simulink library "etherlab_lib_exp"  (Simulink 6.4)
undefined symbols (not defined in the file or in its folder): Address, catch_check
(part 2 of 3)

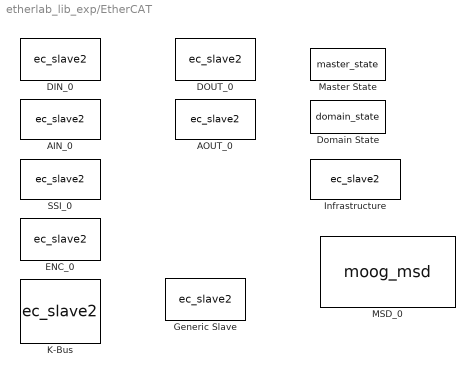
== system etherlab_lib_exp/EtherCAT ==
  AIN_0 : S-Function  FunctionName=ec_slave2  Parameters=Address,SlaveConfig,LayoutVersion,SdoConfig,output,tsample  mask(EL31xx){master=0, index=1, model=EL3102, output_type=Vector Output, scale=1, offset=0, dtype=Double, status=off, filter=off, tau=0.1, tsample=0}
      mask prompts: index "Slave Index"; model "Device Model"; output_type "Output Type"; scale "Output Full Scale"; offset "Output Offset"; dtype "Output Data Type"; status "Status Output"; filter "Output Filter"; tau "LPF Time Constant (sec)"; tsample "Sample Time"
      mask help:
      | Beckhoff 2,4,8-Channel 16-Bit Analog Input
      |
      | Output Type:
      |   1-Byte output: one bit coded input
      |   Vector output: Output vector is <Channels> wide
      |   Separate outputs: have <Channels> number of outputs
      |
      | Input Gain/Offset:
      |   Specify a possible Gain and Offset for the input signal
      mask init:
      | masterStr = '';
      | positionStr = '';
      | [Address masterStr positionStr] = getEtherCATAddress(gcb,master,index);
      | 
      | SdoConfig = [];
      | 
      | % Find the product code from the available models
      | models = struct(...
      |     'EL3102'  ,{{hex2dec('0C1E3052') 0 '-10..10V'}}, ...
      |     'EL3152'  ,{{hex2dec('0C503052') 0 '4..20mA'}}, ...
      |     'EL3162'  ,{{hex2dec('0C5A3052') 0 '0-10V'}} ...  
      |     );
      | 
      | if isfield(models,model)
      |     selection = models.(model);
      | else
      |     errordlg([gcb ': Slave model "' model '" is not implemented'])
      | end
      | 
      | func = selection{3};
      | 
      | EtherCATInfoFile = 'EtherCATInfo_el3xxx';
      | try 
      |     load(EtherCATInfoFile);
      | catch
      |     errordlg([gcb ': Could not load EtherCATInfo MAT file '...
      |         'EtherCATInfo_el3xxx']);
      |     % Regenerate with: 
      |     %  EtherCATInfo_el3xxx = getEtherCATInfo('Beckhoff EL3xxx.xml')
      |     %  save EtherCATInfo_el3xxx 'EtherCATInfo_el3xxx'
      | end
      | LayoutVersion = 0;
      | 
      | output = [];
      | 
      | device = EtherCATInfo_el3xxx(selection{1},selection{2});
      | if isempty(device)
      |     errordlg(sprintf(...
      |         ['%s: Could not find device with\n'...
      |         'ProductCode \t#x%08X\n'...
      |         'RevisionNo \t#x%08X\n'...
      |         'in file %s.'],...
      |         gcs, selection{1}, selection{2}, EtherCATInfoFile));
      | else
      |     channels = str2double(model(6));
      |     if status
      |         StatusPdoEntries = [12544 + (1:channels); ones(1,channels)]';
      |         PdoEntries = [12544 + (1:channels); 1 + ones(1,channels)]';
      |     else
      |         PdoEntries = [25600 + ones(1,channels); 1:channels]';
      |     end
      | 
      |     SlaveConfig = genSlaveConfig(device,EtherCATInfo_el3xxx.VendorId);
      |     PdoEntryMap = generateIO(device);
      |     if output_type == 1
      |         % Vector output chosen
      | 
      |         output(1).PdoEntry = PdoEntries;
      | 
      |         if status
      |             output(2).PdoEntry = StatusPdoEntries;
      |         end
      | 
      |         if dtype ~= 1
      |              output(1).PdoFullScale = 2^15;
      | 
      |             if dtype == 3
      |                 output(1).Gain = scale;
      |                 output(1).Offset = offset;
      |                 output(1).GainName = 'FullScale';
      |                 output(1).OffsetName = 'Offset';
      |             end
      |             if filter
      |                 if sum(tau == 0)
      |                     errordlg([gcb ': Specify a nonzero time constant '...
      |                         'for the output filter.']);
      |                 end
      |                 if (tsample)
      |                     output(1).Filter = tsample./tau;
      |                     output(1).FilterName = 'InputWeight';
      |                 else
      |                     output(1).Filter = 2*pi./tau;
      |                     output(1).FilterName = 'Omega';
      |                 end
      |             end
      |         end
      | 
      |     else
      |         % Separate outputs chosen
      |         % Distribute each row of output_pdo_map to output(x).pdo_map
      |         output = cell2struct(mat2cell(PdoEntries,ones(1,channels),2),'PdoEntry',2);
      |         if status
      |             output = [output; ...
      |                 cell2struct(mat2cell(StatusPdoEntries,ones(1,channels),2),'PdoEntry',2)];
      |         end
      | 
      |         if dtype ~= 1
      |             for i = 1:channels
      |                 output(i).PdoFullScale = 2^15;
      |             end
      | 
      |             if dtype == 3
      |                 if ~isempty(scale)
      |                     for i = 1:channels
      |                         % Choose scale(1) for every output if scale
      |                         % is a scalar
      |                         output(i).Gain = scale(min(i,max(size(scale))));
      |                         output(i).GainName = ['FullScale' num2str(i)];
      |                     end
      |                 end
      | 
      |                 if ~isempty(offset)
      |                     for i = 1:channels
      |                         % Choose offset(1) for every output if offset
      |                         % is a scalar
      |                         output(i).Offset = offset(min(i,max(size(offset))));
      |                         output(i).OffsetName = ['Offset' num2str(i)];
      |                     end
      |                 end
      |             end
      | 
      |             if filter && ~isempty(tau)
      |                 if sum(tau == 0)
      |                     errordlg([gcb ': Specify a nonzero time constant '...
      |                         'for the output filter.']);
      |                 end
      | 
      |                 if tsample(1)
      |                     k = tsample(1)./tau;
      |                     prefix = 'InputWeight';
      |                 else
      |                     k = 2*pi./tau;
      |                     prefix = 'Omega';
      |                 end
      |                 for i = 1:channels
      |                     % Choose k(1) for every output if k
      |                     % is a scalar
      |                     output(i).Filter = k(min(i,max(size(k))));
      |                     output(i).FilterName = [prefix num2str(i)];
      |                 end
      | 
      |             end
      |         end
      |     end
      | end
      mask Help:
      | This block generically implements the EtherCAT 16-Bit Analog Input Terminal for various models.
      | <p/>
      | The following Terminals are supported:
      | <center>
      | <table width="80%">
      | <tr><td>EL3102,4,8</td><td>-10..10V Voltage Input</td></tr>
      | <tr><td>EL3112,4   </td><td>0..20mA Current Input</td></tr>
      | <tr><td>EL3122,4   </td><td>4..20mA Current Input</td></tr>
      | <tr><td>EL3142,4,8</td><td>0..20mA Current Input</td></tr>
      | <tr><td>EL3152,4,8</td><td>4..20mA Current Input</td></tr>
      | <tr><td>EL3162,4,8</td><td>0..10V Voltage Input</td></tr>
      | </table>
      | </center>
      | <p/>
      | Choose and set the following options:
      | <h4>Master:</h4>
      | Set the EtherCAT Master of this terminal.
      | 
      | <h4>Slave Index:</h4>
      | Set the EtherCAT slave index. Following address formats are allowed:
      | <ol>
      | <li> Absolute addressing: a number <<b><tt>n</tt></b>> representing the (zero based) absolute index. <b><tt>n</tt></b> is typically larger than 0 because the first coupler has that address.
      | 
      | <li> Field addressing: Has the form <<b><tt>f:n</tt></b>> where <b><tt>f</tt></b> is the (zero based) EtherCAT coupler field and
      | <b><tt>n</tt></b> is the terminal offset in that field. Take note that <b><tt>n</tt></b> is also greater than 0.
      | 
      | <li> SSId addressing: the Secondary Slave Addressing has the form <<b><tt>#s:n</tt></b>> where <b><tt>s</tt></b> is the Secondary Slave Id of the EtherCAT coupler and <b><tt>n</tt></b> is the offset in that field. The SSId has to be preprogrammed into the coupler with other service tools.
      | </ol>
      | 
      | <h4>Device Model:</h4>
      | Choose the model at the Indexed position of the master.
      | 
      | <h4>Output Type:</h4>
      | <ul>
      | <li>Choose <b>Vector Output</b> to have a single output as a vector
      | with a size corresponding to the channel count of the terminal. This mode also allows a status output port to be displayed. <br/>
      | <li>Choose <b>Separate Outputs</b> to have one output for every channel.
      | </ul>
      | <h4>Output Full Scale</h4>
      | When <b>Output Data Type</b> is set to <b>Double with scale and offset</b>, the block's output value at full scale terminal input can be set here.
      | 
      | <h4>Output Offset</h4>
      | When <b>Output Data Type</b> is set to <b>Double with scale and offset</b>, the blocks output at zero terminal input can be set here. Note that the Full Scale above is also increased by this amount. Note furthermore that this corresponds to the minimum input for terminals such as 4..20mA.
      | 
      | <h4>Output Data Type</h4>
      | Choose the block's output data type for the output signal. Available are:
      | <ul>
      | <li><b><tt>Raw</tt></b> outputting the internal raw value as <tt>int16_T</tt> or <tt>uint16_T</tt> as appropriate
      | <li><b><tt>Double</tt></b> outputting 0..10, -10..10, 0..0.02 and 0.004..0.02 depending on the Model as appropriate
      | <li><b><tt>Double with scale and offset</tt></b>, allowing the output to be scaled with an offset.
      | </ul>
      | 
      | <p>
      | Choosing <b>Status Output</b> provides a port of type <tt>uint8_T</tt> where the status is presented. This is only enabled when <b>Vector Output</b> is selected. Terminal input over- and underrange can be detected using this output. See the terminal's documentation.
      | 
      | <h4>Output Filter</h4>
      | When not in <b>Raw</b> mode, the <b>Output Filter</b> checkbox becomes available, allowing the use of an internal low pass filter. Enter the <b>LPF Time Constant</b> for the filter in the field below.
      | <br>For continuous sample time systems (0 in Sample Time), the filter is also continuous. Discrete samples systems (Sample Time > 0) uses an equivalent discrete low pass filter with a similar time constant.
      | 
      | <p>
      | Set the <b>Sample Time</b> for the block. <tt>0</tt> is continuous sample time (runs at the model's base rate). Setting <tt>-1</tt> will try to set the time using back propagation.
      mask StyleString: edit,edit,popup(EL3102|EL3152|EL3162),popup(Vector Output|Separate Outputs),edit,edit,popup(Raw bits|Double|Double with scale and offset),checkbox,checkbox,edit,edit
      mask CallbackString:
      | |||el31xx_check('output_type');
      | |||el31xx_check('dtype');||el31xx_check('filter');||
      mask Display:
      | fprintf('%s\n%s AIn\nM:%s Idx:%s',...
      |     model,func,masterStr,positionStr)
  AOUT_0 : S-Function  FunctionName=ec_slave2  Parameters=Address,SlaveConfig,LayoutVersion,SdoConfig,input,tsample  mask(EL41xx){master=0, index=1, model=EL4102, input_type=Vector Input, scale=[], tsample=-1}
      mask prompts: index "Slave Index"; model "Device Model"; input_type "Input Type"; scale "Input Full Scale (empty for none)"; tsample "Sample Time (-1 for inherited)"
      mask help:
      | Beckhoff 2,4,8-Channel 16-Bit Analog Output
      |
      | Input Type:
      |   1-Byte input: one bit coded input
      |   Vector input: Input vector is <Channels> wide
      |   Separate inputs: have <Channels> number of inputs
      mask init:
      | masterStr = '';
      | positionStr = '';
      | [Address masterStr positionStr] = getEtherCATAddress(gcb,master,index);
      | 
      | SdoConfig = [];
      | 
      | % Find the product code from the available models
      | models = struct(...
      |     'EL4102'  ,{{hex2dec('10063052') 0                   '0..10V' }}, ...
      |     'EL4132'  ,{{hex2dec('10243052') hex2dec('F0000000') '+-10V'  }}, ...
      |     'EL4132v2',{{hex2dec('10243052') 0                   '+-10V'  }}, ...
      |     'EL4122'  ,{{hex2dec('101a3052') 0                   '4..20mA'}},...  
      |     'EL4112'  ,{{hex2dec('10103052') 0                   '0..20mA'}} ...  
      |     );
      | 
      | SdoConfig = [];
      | 
      | if isfield(models,model)
      |     selection = models.(model);
      | else
      |     errordlg([gcb ': Slave model "' model '" is not implemented'])
      | end
      | 
      | func = selection{3};
      | 
      | EtherCATInfoFile = 'EtherCATInfo_el4xxx';
      | try 
      |     load(EtherCATInfoFile);
      | catch
      |     errordlg([gcb ': Could not load EtherCATInfo MAT file '...
      |         'EtherCATInfo_el4xxx']);
      |     % Regenerate with: 
      |     %  EtherCATInfo_el4xxx = getEtherCATInfo('Beckhoff EL4xxx.xml')
      |     % Note that in this case you will not have Rev #xF0000000 for
      |     % EL4132 then, unless you create one yourself
      | end
      | 
      | LayoutVersion = 0;
      | 
      | device = EtherCATInfo_el4xxx(selection{1},selection{2});
      | input = [];
      | if isempty(device)
      |     errordlg(sprintf(...
      |         ['%s: Could not find device with\n'...
      |         'ProductCode \t#x%08X\n'...
      |         'RevisionNo \t#x%08X\n'...
      |         'in file %s.'],...
      |         gcs, selection{1}, selection{2}, EtherCATInfoFile));
      | else
      |     SlaveConfig = genSlaveConfig(device, EtherCATInfo_el4xxx.VendorId);
      |     % Number of channels is given by the 6'th character of model string
      |     channels = str2double(model(6));
      | 
      |     input = [];
      |     if input_type == 1
      |         PdoEntryMap = generateIO(device, 'GroupType', 'All');
      |         input = cell2struct(PdoEntryMap,'PdoEntry',1);
      |         input.PdoFullScale = 2^15;
      |         if ~isempty(scale)
      |             input.Gain = scale;
      |             input.GainName = 'FullScale';
      |         end
      |     elseif input_type == 2
      |         PdoEntryMap = generateIO(device);
      |         fs = repmat({2^15},1,channels);
      |         input = struct('PdoEntry', PdoEntryMap, 'PdoFullScale', 2^15);
      |         if ~isempty(scale)
      |             for i = 1:channels
      |                 input(i).Gain = scale(min(i,max(size(scale))));
      |                 input(i).GainName = ['FullScale' num2str(i)];
      |             end
      |         end
      |     end
      | end
      mask Help:
      | This block generically implements the EtherCAT 16-Bit Analog Input Terminal for various models.
      | <p/>
      | The block input is generally a <tt>double</tt> corresponding the the terminal's capability. Thus a 4..20mA terminal expects values in the range [0.004..0.02). If a digital input is required, only <tt>uint16</tt> or <tt>int16</tt> is accepted, depending on whether the the terminal is bipolar or not.
      | <p/>
      | Exceeding the input range simply saturates the terminal's output.
      | <p/>
      | The following Terminals are supported:
      | <center>
      | <table width="80%">
      | <tr><td>EL4102,4,8</td><td>0..10V Voltage Output</td></tr>
      | <tr><td>EL4112,4,8</td><td>0..20mA Current Output</td></tr>
      | <tr><td>EL4122,4,8</td><td>4..20mA Current Output</td></tr>
      | <tr><td>EL4132,4,8</td><td>-10..10V Voltage Output</td></tr>
      | </table>
      | </center>
      | <p/>
      | Choose and set the following options:
      | <h4>Master:</h4>
      | Set the EtherCAT Master of this terminal.
      | 
      | <h4>Slave Index:</h4>
      | Set the EtherCAT slave index. Following address formats are allowed:
      | <ol>
      | <li> Absolute addressing: a number <<b><tt>n</tt></b>> representing the (zero based) absolute index. <b><tt>n</tt></b> is typically larger than 0 because the first coupler has that address.
      | 
      | <li> Field addressing: Has the form <<b><tt>f:n</tt></b>> where <b><tt>f</tt></b> is the (zero based) EtherCAT coupler field and
      | <b><tt>n</tt></b> is the terminal offset in that field. Take note that <b><tt>n</tt></b> is also greater than 0.
      | 
      | <li> SSId addressing: the Secondary Slave Addressing has the form <<b><tt>#s:n</tt></b>> where <b><tt>s</tt></b> is the Secondary Slave Id of the EtherCAT coupler and <b><tt>n</tt></b> is the offset in that field. The SSId has to be preprogrammed into the coupler with other service tools.
      | </ol>
      | 
      | <h4>Device Model:</h4>
      | Choose the device at the Indexed position of the master.
      | 
      | <h4>Input Type:</h4>
      | <ul>
      | <li>Choose <b>Vector Input</b> to have a single input as a vector
      | with a size corresponding to the channel count of the terminal. This mode also allows a control input and a status output port to be displayed.
      | <li>Choose <b>Separate Inputs</b> to have one input for every channel.
      | </ul>
      | 
      | <p>
      | Choosing <b>Status Output</b> provides a port of type <tt>uint8_T</tt> where the status is presented. This is only enabled when <b>Vector Output</b> is selected. Note: at the time of writing (1.2.2006) the terminals do not have a status output, and hence this option is disabled!
      | 
      | <p>
      | Set the <b>Sample Time</b> for the block. <tt>0</tt> is continuous sample time (runs at the model's base rate). Setting <tt>-1</tt> will try to set the time using back propagation.
      mask StyleString: edit,edit,popup(EL4102|EL4112|EL4122|EL4132v2|-- Obsolete|EL4132),popup(Vector Input|Separate Inputs),edit,edit
      mask Display:
      | fprintf('%s\n%s AIn\nM:%s Idx:%s',...
      |     model,func,masterStr,positionStr)
  DIN_0 : S-Function  FunctionName=ec_slave2  Parameters=Address,SlaveConfig,LayoutVersion,SdoConfig,IOSpec,tsample  mask(EL10xx){master=0, index=1, model=EL1004v2, output_type=Vector Output, tsample=0}
      mask prompts: index "Slave Index"; model "Device Model"; output_type "Output Type"; tsample "Sample Time"
      mask help:
      | Beckhoff EtherCAT Digital Input
      | EL1002,4,8:	3ms filter
      | EL1012,4,8:	10us filter
      | EL1004v2: Newer version with PDO at 0x6000
      |
      | Output Type:
      |   1-Byte output: one bit coded output
      |   Vector output: Output vector is <Channels> wide
      |   Separate outputs: have <Channels> number of outputs
      mask init:
      | masterStr = '';
      | positionStr = '';
      | [Address masterStr positionStr] = getEtherCATAddress(gcb,master,index);
      | 
      | SdoConfig = [];
      | 
      | % Find the product code from the available models
      | models = struct(...
      |     'EL1004'  ,[hex2dec('03ec3052')     hex2dec('0010000A')], ...
      |     'EL1004v2',[hex2dec('03ec3052')     hex2dec('00100000')], ...
      |     'EL1008'  ,[hex2dec('03f03052')     hex2dec('00100000')], ...
      |     'EL1014v2',[hex2dec('03f63052')     hex2dec('00100000')], ...  
      |     'EL1014'  ,[hex2dec('03f63052')     hex2dec('00000000')], ...  
      |     'EL1018'  ,[hex2dec('03fa3052')     hex2dec('00100000')]  ...
      |     );
      | 
      | if isfield(models,model)
      |     selection = models.(model);
      | else
      |     errordlg([gcb ': Slave model "' model '" is not implemented'])
      | end
      | 
      | EtherCATInfoFile = 'EtherCATInfo_el1xxx';
      | try 
      |     load(EtherCATInfoFile);
      | catch
      |     errordlg([gcb ': Could not load EtherCATInfo MAT file '...
      |         'EtherCATInfo_el1xxx']);
      |     % Regenerate with: 
      |     %  EtherCATInfo_el1xxx = getEtherCATInfo('Beckhoff EL1xxx.xml')
      |     %  save EtherCATInfo_el1xxx
      | end
      | 
      | LayoutVersion = 0;
      | 
      | IOSpec = [];
      | 
      | device = EtherCATInfo_el1xxx(selection(1),selection(2));
      | if isempty(device)
      |     errordlg(sprintf(...
      |         ['%s: Could not find device with\n'...
      |         'ProductCode \t#x%08X\n'...
      |         'RevisionNo \t#x%08X\n'...
      |         'in file %s.'],...
      |         gcs, selection(1), selection(2), EtherCATInfoFile));
      | else
      |     
      |     SlaveConfig = ...
      |         genSlaveConfig(device,EtherCATInfo_el1xxx.VendorId);
      |     
      |     if strcmp(output_type, 'Vector Output')
      |         % Only one output, with all rows of pdo_map
      |         PdoEntryMap = generateIO(device, 'GroupType', 'All');
      |         IOSpec = cell2struct(PdoEntryMap,'PdoEntry',1);
      | 
      |     elseif strcmp(output_type, 'Separate Outputs')
      |         % Have (channel) number of outputs, each containing one row of pdo_map
      |         PdoEntryMap = generateIO(device);
      |         IOSpec = cell2struct(PdoEntryMap,'PdoEntry',1);
      |     else
      |         errordlg([gcb ': unknown output type: ' output_type]);
      |         IOSpec = [];
      |     end
      | end
      mask Help:
      | This block implements the Beckhoff's EtherCAT series of Digital Input Terminals.
      | <p/>
      | Choose or set the following options:
      | <h4>Master:</h4>
      | Set the EtherCAT Master number that this terminal is connected to.
      | 
      | <h4>Slave Index:</h4>
      | Set the EtherCAT slave index. Following address formats are allowed:
      | <ol>
      | <li> Absolute addressing: a number <<b><tt>n</tt></b>> representing the (zero based) absolute index. <b><tt>n</tt></b> is typically larger than 0 because the first coupler has that address.
      | 
      | <li> Field addressing: Has the form <<b><tt>f:n</tt></b>> where <b><tt>f</tt></b> is the (zero based) EtherCAT coupler field and
      | <b><tt>n</tt></b> is the terminal offset in that field. Take note that <b><tt>n</tt></b> is also greater than 0.
      | 
      | <li> SSId addressing: the Secondary Slave Addressing has the form <<b><tt>#s:n</tt></b>> where <b><tt>s</tt></b> is the Secondary Slave Id of the EtherCAT coupler and <b><tt>n</tt></b> is the offset in that field. The SSId has to be preprogrammed into the coupler with other service tools.
      | </ol>
      | 
      | <h4> Device Model</h4>
      | Select the model that is used. This sets the number of outputs of this block.
      | 
      | <h4>Output Type</h4>
      | The block output type corresponding to the terminal inputs can be one of the following:
      | <ul>
      | <li><b>1-Byte Output</b>: This sets one output where each digital input to the terminal occupies one bit.
      | <li><b>Vector Output</b>: This sets one output vector with a width equal to the number of digital inputs to the terminal.
      | <li><b>Separate Outputs</b>: This sets the number of outputs corresponding to the digital inputs to the terminal.
      | </ul>
      | 
      | <h4>Output Data Type</h4>
      | Select the output data type that is required.
      | 
      | <h4>Sample Time</h4>
      | Select the correct sample time. Setting this to 0 makes for a sample time at the model's base rate. If another block can set the sample time, choose -1 for inherited sample time.
      mask StyleString: edit,edit,popup(EL1004v2|EL1008|EL1014v2|EL1018|-- Obsolete|EL1004|EL1014),popup(Vector Output|Separate Outputs),edit
      mask Display:
      | fprintf('%s\nM:%s Idx:%s',...
      |     model,'',positionStr)
  DOUT_0 : S-Function  FunctionName=ec_slave2  Parameters=Address,SlaveConfig,LayoutVersion,SdoConfig,IOSpec,tsample  mask(EL20xx){master=0, index=1, model=EL2004v2, input_type=Vector Input, status=off, tsample=0}
      mask prompts: index "Slave Index"; model "Device Model"; input_type "Input Type"; status "Status Output"; tsample "Sample Time (-1 for inherited)"
      mask help:
      | Beckhoff EtherCAT Digital Output
      | EL2002,4:	24V 0.5A
      | EL2032:		24V 2A, Optional Status (with Vector Input)
      |
      | Input Type:
      |   1-Byte input: one bit coded input
      |   Vector input: Input vector is <Channels> wide
      |   Separate inputs: have <Channels> number of inputs
      mask init:
      | masterStr = '';
      | positionStr = '';
      | [Address masterStr positionStr] = getEtherCATAddress(gcb,master,index);
      | 
      | SdoConfig = [];
      | 
      | % Find the product code from the available models
      | models = struct(...
      |     'EL2004'  ,[hex2dec('07d43052')  hex2dec('00000000')], ...
      |     'EL2004v2',[hex2dec('07d43052')  hex2dec('00100000')], ...
      |     'EL2008'  ,[hex2dec('07d83052')  hex2dec('00100000')], ...
      |     'EL2032'  ,[hex2dec('07f03052')  hex2dec('00000000')], ...
      |     'EL2032v2',[hex2dec('07f03052')  hex2dec('00100000')], ...
      |     'EL2602'  ,[hex2dec('0a2a3052')  hex2dec('00100000')], ...
      |     'EL2612'  ,[hex2dec('0a343052')  hex2dec('00100000')], ...
      |     'EL2622'  ,[hex2dec('0a3e3052')  hex2dec('00100000')]  ...
      |     );
      | 
      | if isfield(models,model)
      |     selection = models.(model);
      | else
      |     errordlg([gcb ': Slave model "' model '" is not implemented'])
      | end
      | 
      | LayoutVersion = 0;
      | 
      | try 
      |     load EtherCATInfo_el2xxx;
      | catch
      |     errordlg([gcb ': Could not load EtherCATInfo MAT file '...
      |         'EtherCATInfo_el2xxx']);
      |     % Regenerate with: 
      |     %  EtherCATInfo_el2xxx = getEtherCATInfo('Beckhoff EL2xxx.xml')
      |     %  save EtherCATInfo_el2xxx 'EtherCATInfo_el2xxx'
      | end
      | 
      | IOSpec = [];
      | 
      | device = EtherCATInfo_el2xxx(selection(1),selection(2));
      | if isempty(device)
      |     errordlg(sprintf(...
      |         ['%s: Could not find device with\n'...
      |         'ProductCode \t#x%08X\n'...
      |         'RevisionNo \t#x%08X\n'...
      |         'in file "%s".'],...
      |         gcs, selection(1), selection(2), 'EtherCATInfo_el2xxx'));
      | else
      |     SlaveConfig = genSlaveConfig(device,EtherCATInfo_el2xxx.VendorId);
      |     
      |     channels = str2double(model(6));
      |     PdoIndexList = hex2dec('1600') + [0:channels-1];
      |     if status
      |         PdoIndexList = [PdoIndexList  hex2dec('1A00') + [0:channels-1]];
      |     end
      | 
      |     if strcmp(input_type,'Vector Input')
      |         % Only one output, with all rows of pdo_map
      |         PdoEntryMap = generateIO(device, 'GroupType', 'All',...
      |             'SelectPdo', PdoIndexList);
      |         IOSpec = cell2struct(PdoEntryMap,'PdoEntry',1);
      |     elseif strcmp(input_type, 'Separate Inputs')
      |         % Have (channel) number of outputs, each containing one row of pdo_map
      |         PdoEntryMap = generateIO(device);
      |         IOSpec = cell2struct(PdoEntryMap,'PdoEntry',1);
      |     else
      |         errordlg([gcb ': unknown input type: ' input_type]);
      |     end
      | end
      mask Help:
      | This block implements the Beckhoff's EtherCAT series of Digital Output Terminals.
      | <p/>
      | Choose or set the following options:
      | <h4>Master:</h4>
      | Set the EtherCAT Master number that this terminal is connected to.
      | 
      | <h4>Slave Index:</h4>
      | Set the EtherCAT slave index. Following address formats are allowed:
      | <ol>
      | <li> Absolute addressing: a number <<b><tt>n</tt></b>> representing the (zero based) absolute index. <b><tt>n</tt></b> is typically larger than 0 because the first coupler has that address.
      | 
      | <li> Field addressing: Has the form <<b><tt>f:n</tt></b>> where <b><tt>f</tt></b> is the (zero based) EtherCAT coupler field and
      | <b><tt>n</tt></b> is the terminal offset in that field. Take note that <b><tt>n</tt></b> is also greater than 0.
      | 
      | <li> SSId addressing: the Secondary Slave Addressing has the form <<b><tt>#s:n</tt></b>> where <b><tt>s</tt></b> is the Secondary Slave Id of the EtherCAT coupler and <b><tt>n</tt></b> is the offset in that field. The SSId has to be preprogrammed into the coupler with other service tools.
      | </ol>
      | 
      | <h4> Device Model</h4>
      | Select the model that is used. This sets the maximum number of inputs of this block. Having fewer inputs is allowed.<br>
      |  Some models have an optional status byte. These have the <b>Status Output</b> below enabled.
      | 
      | <h4>Input Type</h4>
      | The input type can be one of the following:
      | <ul>
      | <li><b>1-Byte Input</b>: This sets one block input bit coded corresponding to the digital output of the terminal.
      | <li><b>Vector Input</b>: This sets one input vector where each element corresponds to a digital output of the terminal.
      | <li><b>Separate Inputs</b>: This sets the number of block inputs corresponding to the digital output count of the terminal.
      | </ul>
      | 
      | <h4>Status Output</h4>
      | Some models have a status bit to monitor the attached hardware. Check this box to make it available as a block output in simulink. This option is not available if <b>Separate Inputs</b> is selected.
      | 
      | <h4>Sample Time</h4>
      | Select the correct sample time. Setting this to 0 makes for a sample time at the model's base rate. If another block can set the sample time, choose -1 for inherited sample time.
      mask StyleString: edit,edit,popup(EL2004v2|EL2008|EL2032v2|EL2602|EL2612|EL2622|-- Obsolete|EL2004|EL2032),popup(Vector Input|Separate Inputs),checkbox,edit
      mask CallbackString:
      | ||status_idx = find(strcmp(get_param(gcb,'MaskNames'),'status'));
      | 
      | en = get_param(gcb,'MaskEnables');
      | 
      | if findstr('2032',get_param(gcb,'model'))
      |         en{status_idx} = 'on';
      | else
      |     en{status_idx} = 'off';
      | end
      | set_param(gcb,'MaskEnables',en);
      | |||
      mask Display:
      | fprintf('%s\nM:%s Idx:%s',...
      |     model,masterStr,positionStr)
  Domain State : S-Function  FunctionName=domain_state  Parameters=master,domain,input,output,tsample  mask(Domain State){master=0, domain=0, direction=Input Only, tsample=0}
      mask prompts: tsample "Sample Time"
      mask help:
      | Displays the following domain state information:
      | * Working Counter
      | * Domain state:
      | 	0 - No slaves
      | 	1 - Domain incomplete
      | 	2 - Domain complete
      mask init:
      | switch direction
      |     case 1
      |         input = 1;
      |         output = 0;
      |     case 2
      |         input = 0;
      |         output = 1;
      |     case 3
      |         input = 1;
      |         output = 1;
      | end
      mask StyleString: edit,edit,popup(Input Only|Output Only|Input and Output),edit
      mask Display:
      | fprintf('Domain State\nM:%u d:%u',
      | master,domain);
  ENC_0 : S-Function  FunctionName=ec_slave2  Parameters=Address,SlaveConfig,LayoutVersion,SdoConfig,IOSpec,tsample  mask(EL5101){master=0, index=1, reload=off, reset=off, fwdcount=off, gate=None, freqwin=100, reloadvalue=65535, control=off, preset=off, dtype=Double, value=on, latch=off, freq=off, period=off, window=off, status=off, tsample=0}
      mask prompts: index "Slave Index"; reload "Enable Register Reload"; reset "Enable Index Reset"; fwdcount "Enable FWD Count"; freqwin "Frequency Window (0..65535)"; reloadvalue "Counter Reload Value (0..65535)"; control "Control Input Port"; preset "Preset Input Port"; dtype "Output Data Type"; value "Counter Value Output Port"; latch "Latch Output Port"; freq "Frequency Output Port"; period "Period Output Port"; window "Window Output Port"; status "Status Output Port"; tsample "Sample Time (-1 inherited)"
      mask help: Beckhoff EtherCAT Incremental Encoder Input
      mask init:
      | masterStr = '';
      | positionStr = '';
      | [Address masterStr positionStr] = getEtherCATAddress(gcb,master,index);
      | 
      | product_code = hex2dec('13ed3052');
      | revision_no = hex2dec('00010000');
      | LayoutVersion = 0;
      | 
      | try 
      |     load EtherCATInfo_el5xxx
      | catch
      |     errordlg([gcb ': Could not load EtherCATInfo MAT file '...
      |         'EtherCATInfo_el5xxx']);
      |     % Regenerate with: 
      |     %  EtherCATInfo_el5xxx = getEtherCATInfo('Beckhoff EL5xxx.xml')
      |     %  save EtherCATInfo_el5xxx 'EtherCATInfo_el5xxx'
      | end
      | SlaveConfig = genSlaveConfig(EtherCATInfo_el5xxx, product_code, revision_no);
      | 
      | 
      | % PDO Entry is a definition of all PDO's that exist in the slave
      | % List here a matrix, where every row has 3 elements:
      | % 1: PDO index
      | % 2: PDO subindex
      | % 3: Bit size (8,16,32); Negative values mean signed values
      | pdo_entry = struct(...
      |     'status' , [hex2dec('6000'), 1], ...
      |     'value'  , [hex2dec('6000'), 2], ...
      |     'latch'  , [hex2dec('6000'), 3], ...
      |     'freq'   , [hex2dec('6000'), 4], ...
      |     'period' , [hex2dec('6000'), 5], ...
      |     'window' , [hex2dec('6000'), 6], ...
      |     'control', [hex2dec('7000'), 1], ...
      |     'preset' , [hex2dec('7000'), 2]);
      | 
      | 
      | % SDO Config is the configuration of a slave
      | % It is a matrix, every row having 4 elements:
      | % 1: SDO Index
      | % 2: SDO Subindex
      | % 3: Size    (8,16,32)
      | % 4: value
      | SdoConfig = [
      |     hex2dec('8000'), 1,  8, reloadvalue == 1;... % Reload
      |     hex2dec('8000'), 2,  8, reset == 1      ;... % Index Reset
      |     hex2dec('8000'), 3,  8, fwdcount == 1   ;... % Forward Count
      |     hex2dec('8000'), 4,  8, gate == 2       ;... % Positive Gate
      |     hex2dec('8000'), 5,  8, gate == 3       ;... % Negative Gate
      |     hex2dec('8001'), 1, 16, freqwin         ;... % Frequency Window
      |     hex2dec('8001'), 2, 16, reloadvalue     ;... % Reload Value
      |     ];
      | SdoConfig = cell2struct(...
      |     num2cell(SdoConfig),...
      |     {'Index' 'SubIndex' 'BitLen' 'Value'}, 2);
      | 
      | % This maps ???
      | % It is a matrix, every row having 4 elements:
      | % 1: PDO direction as seen by the slave: 0 = output; 1 = Input
      | % 2: PDO Index
      | % 3: Starting row of PDO entry (Zero based)
      | % 4: Number of PDO entry rows
      | IOSpec = [];
      | if ~isempty(SlaveConfig)
      |     port = 1;
      |     if value
      |         IOSpec(port).PdoEntry = pdo_entry.value;
      |         if dtype == 2
      |             IOSpec(port).PdoFullScale = 2^16;
      |         end
      | 
      |         port = port + 1;
      |     end
      |     if latch
      |         IOSpec(port).PdoEntry = pdo_entry.latch;
      |         if dtype == 2
      |             IOSpec(port).PdoFullScale = 2^16;
      |         end
      | 
      |         port = port + 1;
      |     end
      |     if freq
      |         IOSpec(port).PdoEntry = pdo_entry.freq;
      |         if dtype == 2
      |             IOSpec(port).PdoFullScale = 2^32;
      |         end
      | 
      |         port = port + 1;
      |     end
      |     if period
      |         IOSpec(port).PdoEntry = pdo_entry.period;
      |         if dtype == 2
      |             IOSpec(port).PdoFullScale = 2^16;
      |         end
      | 
      |         port = port + 1;
      |     end
      |     if window
      |         IOSpec(port).PdoEntry = pdo_entry.window;
      |         if dtype == 2
      |             IOSpec(port).PdoFullScale = 2^16;
      |         end
      | 
      |         port = port + 1;
      |     end
      |     if status
      |         IOSpec(port).PdoEntry = pdo_entry.status;
      | 
      |         port = port + 1;
      |     end
      | 
      |     if control
      |         IOSpec(port).PdoEntry = pdo_entry.control;
      | 
      |         port = port + 1;
      |     end
      |     if preset
      |         IOSpec(port).PdoEntry = pdo_entry.preset;
      |         if dtype == 2
      |             IOSpec(port).PdoFullScale = 2^16;
      |         end
      | 
      |         port = port + 1;
      |     end
      | end
      mask Help:
      | This block implements the EtherCAT Incremental Encoder Input Terminal EL5101.
      | 
      | The first output is data, the second optional output is a Status Byte. Various options affect the behaviour of the terminal and the block's output:
      | 
      | <h4>Master:</h4>
      | Set the EtherCAT Master of this terminal.
      | 
      | <h4>Slave Index:</h4>
      | Set the EtherCAT slave index. Following address formats are allowed:
      | <ol>
      | <li> Absolute addressing: a string '<b><tt>n</tt></b>' representing the (zero based) absolute index. <b><tt>n</tt></b> is typically larger than 0 because the first coupler has that address.
      | 
      | <li> SSId addressing: the Secondary Slave Addressing has the form '<b><tt>#s:n</tt></b>' where <b><tt>s</tt></b> is the Secondary Slave Id of the EtherCAT coupler and <b><tt>n</tt></b> is the offset in that field. The SSId has to be preprogrammed into the coupler with other service tools.
      | </ol>
      | 
      | <h4>Configuration Parameters</h4>
      | <dl>
      | <dt><b><tt>Enable Register Reload</tt></b></dt>
      | <dd>When the counter value wraps (either overflows or underflows), reload the value specified in <em>Counter Reload Value</em>. This option cannot be used together with <em>Enable Index Reset</em></dd>
      | 
      | <dt><b><tt>Enable Index Reset</tt></b></dt>
      | <dd>activates terminal input "C", which resets the counter value. This option cannot be used together with <em>Enable Register Reload</em>.</dd>
      | 
      | <dt><b><tt>Enable FWD Count</tt></b></dt>
      | <dd>disables quadrature evaluation of the "A" and "B" terminal inputs. Counter only counts up.</dd>
      | 
      | <dt><b><tt>Gate</tt></b></dt>
      | <dd>
      | Stops the counter on either <b>Rising</b> or <b>Falling</b> edge. This input is enabled when <em>Latch Output Port</en> is enabled.
      | </dd>
      | 
      | <dt><b><tt>Frequency Window</tt></b></dt>
      | <dd>Value determines the width of the Window variable in increments of 16us (whatever that means???) This input is enabled when <em>Frequency Output Port</em> is selected</dd>
      | 
      | <dt><b><tt>Counter Reload Value</tt></b></dt>
      | <dd>The value with which the counter is reloaded in case of <em>Enable Register Reload</em> is activated</dd>
      | </dl>
      | 
      | <h4>Inputs</h4>
      | Enable <tt><b>Control Input Port</b></tt> or <tt><b>Preset Input Port</b></tt>. Refer to the documentation for these rather complex inputs. The ordering of the inputs matches the ordering in the configuration mask.
      | 
      | <h4>Output Data Type</h4>
      | Choose the block's output data type for the output signal. Available are:
      | <ul>
      | <li><b><tt>Raw</tt></b> outputting the internal raw value as <tt>uint32_T</tt> as appropriate
      | <li><b><tt>Double</tt></b> outputting 0..1 corresponding to the Full Scale. Full Scale is affected by the Frame Type, SSI Frame Size and Data Length. Refer to manufactuer's documentation.
      | </ul>
      | 
      | <h4>Outputs</h4>
      | Select the desired outputs as presented int the configuratoin mask. The ordering matches the ordering in the mask. Refer to manufacturors documentation.
      | 
      | <p>
      | Set the <b>Sample Time</b> for the block. <tt>0</tt> is continuous sample time (runs at the model's base rate). Setting <tt>-1</tt> will try to set the time using back propagation.
      mask StyleString: edit,edit,checkbox,checkbox,checkbox,popup(None|Positive|Negative),edit,edit,checkbox,checkbox,popup(Raw bits|Double),checkbox,checkbox,checkbox,checkbox,checkbox,checkbox,edit
      mask CallbackString: ||el5101_check('Reload');|el5101_check('IndexReset');|||||||||el5101_check('Latch');|el5101_check('Freq');||||
      mask Display:
      | fprintf('EL5101\nIncr.-Enc\nM:%s Idx:%s',...
      |     masterStr, positionStr)
  Generic Slave : S-Function  FunctionName=ec_slave2  Parameters=Address,SlaveConfig,LayoutVersion,SdoConfig,IOSpec,tsample  mask(Generic EtherCAT Slave){master=0, index=1, ethercatinfo='', product_code=hex2dec('0'), revision=[], pdo_list=[], group=No Grouping, sdo_config=[], tsample=0}
      mask prompts: index "Slave Index"; ethercatinfo "EtherCATInfo XML file"; product_code "Product Code"; revision "Revision (empty for latest)"; pdo_list "Mapped PDO (empty for all)"; group "Group PDO Entries"; sdo_config "SDO Config"; tsample "Sample Time (-1 inherited)"
      mask help: Implements a generic EtherCAT Slave as described in the EtherCATInfo XML File
      mask init:
      | masterStr = '';
      | positionStr = '';
      | product_name = 'Unknown';
      | [Address masterStr positionStr] = getEtherCATAddress(gcb,master,index);
      | 
      | SdoConfig = [];
      | 
      | % Generate a LayoutVersion that is unique for every slave
      | % of this type to enure that a separate slave config is generated
      | % for every slave
      | LayoutVersion = 0;
      | 
      | try
      |     fname = char(ethercatinfo);
      | catch
      |     errordlg([gcb ':File name for EtherCAT Info not a valid string']);
      | end
      | 
      | if ~(isnumeric(product_code) && isnumeric(revision) ...
      |         && isnumeric(pdo_list) && isnumeric(sdo_config))
      |     fname = '';
      |     errordlg([gcb ':Value for Product Code, Revision Number '...
      |         'Pdo List and Sdo Config must be numeric']);
      | end
      |     
      | IOSpec = [];
      | SlaveConfig = [];
      | 
      | if isempty(fname)
      |     IOSpec = [];
      |     SlaveConfig = [];
      | elseif isempty(dir(fname))
      |     warndlg([gcb ':File ''' fname ''' not found']);
      | else
      |     switch lower(group)
      |         case 'group data types in pdo'
      |             type = 'PDO';
      |         case 'group data types'
      |             type = 'ALL';
      |         otherwise
      |             type = 'None';
      |     end
      |     ei = EtherCATInfo(fname);
      |     if ~isempty(product_code) && product_code
      |         dev = ei(product_code,revision);
      |     else
      |         dev = ei{1};
      |     end
      |     SlaveConfig = genSlaveConfig(dev, ei.VendorId);
      |     PdoEntries = generateIO(dev,'GroupType',type);
      |     if ~isempty(SlaveConfig)
      |         product_name = SlaveConfig.Type;
      |     end
      |     IOSpec = struct('PdoEntry', PdoEntries);
      | end
      mask StyleString: edit,edit,edit,edit,edit,edit,popup(No Grouping|Group Data Types in PDO|Group Data Types),edit,edit
      mask Display:
      | fprintf('%s\nM:%s Idx:%s',...
      |     product_name,masterStr,positionStr);
  Infrastructure : S-Function  FunctionName=ec_slave2  Parameters=Address,SlaveConfig,LayoutVersion,SdoConfig,output,tsample  mask(Infrastructure Block){master=0, index=0, model=EK1100, tsample=0}
      mask prompts: index "Slave Index"; model "Device Model"; tsample "Sample Time (-1 inherited)"
      mask help:
      | EtherCAT Infrastructure Slaves.
      |
      | The following slaves are available:
      | EK1100	'EtherCAT Coupler
      | EK1110	EtherCAT Extension
      | EL9110	24V w. Diag.
      | EL9160	230V w. Diag.
      | EL9210	24V w. Fuse & Diag.
      | EL9260	230V w. Fuse & Diag.
      |
      | Including these slaves (even if they don't have outputs)
      | in the bus configuration will cause them to go into the
      | operational mode
      mask init:
      | masterStr = '';
      | positionStr = '';
      | [Address masterStr positionStr] = getEtherCATAddress(gcb,master,index);
      | 
      | SdoConfig = [];
      | func = 'Unknown';
      | 
      | % Find the product code from the available models
      | models = struct( ...
      |     'EK1100', {{hex2dec('044c2c52') hex2dec('00000000') 'EtherCAT Coupler'    }}, ...
      |     'EK1110', {{hex2dec('04562c52') hex2dec('00000000') 'EtherCAT Extension'  }}, ...
      |     'EL9110', {{hex2dec('23963052') hex2dec('00100000') '24V w. Diag.'        }}, ...
      |     'EL9160', {{hex2dec('23c83052') hex2dec('00100000') '230V w. Diag.'       }}, ...
      |     'EL9210', {{hex2dec('23fa3052') hex2dec('00100000') '24V w. Fuse & Diag.' }}, ...
      |     'EL9260', {{hex2dec('242c3052') hex2dec('00100000') '230V w. Fuse & Diag.'}} ...
      |     );
      | 
      | if isfield(models,model)
      |     selection = models.(model);
      |     func = selection{3};
      | else
      |     errordlg([gcb ': Slave model "' model '" is not implemented'])
      | end
      | 
      | try
      |     switch model(1:2)
      |         case 'EK'
      |             EtherCATInfoFile = 'EtherCATInfo_ekxxxx';
      |             load(EtherCATInfoFile);
      |             ei = EtherCATInfo_ekxxxx;
      |         case 'EL'
      |             EtherCATInfoFile = 'EtherCATInfo_el9xxx';
      |             load(EtherCATInfoFile);
      |             ei = EtherCATInfo_el9xxx;
      |     end
      | catch
      |     errordlg([gcb ': Could not load EtherCATInfo MAT file ' EtherCATInfoFile]);
      | end
      | LayoutVersion = 0;
      | 
      | output = [];
      | dev = ei(selection{1}, selection{2});
      | SlaveConfig = genSlaveConfig(dev,ei.VendorId);
      | if ~isempty(dev)
      |     PdoEntries = generateIO(dev);
      |     output = struct('PdoEntry',PdoEntries);
      | end
      mask StyleString: edit,edit,popup(EK1100|EK1110|EL9110|EL9160|EL9210|EL9260),edit
      mask Display:
      | fprintf('%s\n%s\nM:%s Idx:%s',...
      |     model,func,masterStr,positionStr)
  K-Bus : S-Function  FunctionName=ec_slave2  Parameters=Address,SlaveConfig,LayoutVersion,SdoConfig,IOSpec,tsample  mask(K-Bus Coupler){master=0, index=1, ethercatinfo='', group=Group Data Types in PDO, tsample=0}
      mask prompts: index "Slave Index"; ethercatinfo "EtherCATInfo XML file"; group "Group Pdo Entries"; tsample "Sample Time (-1 inherited)"
      mask help:
      | Beckhoff EK1110 K-Bus to EtherCAT Coupler
      |
      | Group Pdo Entries:
      |   * Data Types in PDO: This option groups all Pdo Entries in a
      | 	PDO with the same data type together
      |   * All Data Types: All Pdo Entries with the same data typ
      | 	are grouped together.
      mask init:
      | masterStr = '';
      | positionStr = '';
      | display_name = '';
      | [Address masterStr positionStr] = getEtherCATAddress(gcb,master,index);
      | 
      | SdoConfig = [];
      | 
      | % Generate a LayoutVersion that is unique for every slave
      | % of this type to enure that a separate slave config is generated
      | % for every slave
      | LayoutVersion = Address.Domain * 2^16 + Address.Position;
      | 
      | fname = '';
      | 
      | try
      |     fname = char(ethercatinfo);
      | catch
      |     errordlg([gcb ':File name for EtherCAT Info not a valid string']);
      | end
      |     
      | IOSpec = [];
      | SlaveConfig = [];
      | 
      | if isempty(fname)
      |     IOSpec = [];
      |     SlaveConfig = [];
      | elseif isempty(dir(fname))
      |     warndlg([gcb ':File ''' fname ''' not found']);
      | else
      |     switch lower(group)
      |         case 'group data types in pdo'
      |             type = 'PDO';
      |         case 'group data types'
      |             type = 'ALL';
      |         otherwise
      |             type = 'None';
      |     end
      |     
      |     ei = EtherCATInfo(fname);
      |     SlaveConfig = genSlaveConfig(ei{1},ei.VendorId);
      |     PdoEntries = generateIO(ei{1},'GroupType',type);
      |     IOSpec = struct('PdoEntry', PdoEntries);
      | 
      |     [p f e] = fileparts(fname);
      |     display_name = [f e];
      | end
      mask Help:
      | This block provides an interface to the K-Bus process image for the EK1120 Coupler.
      | <p>
      | Choose and set the following options:
      | <h4>Master:</h4>
      | Set the EtherCAT Master of this terminal.
      | 
      | <h4>Slave Index:</h4>
      | Set the EtherCAT slave index. Following address formats are allowed:
      | <ol>
      | <li> Absolute addressing: a string '<b><tt>n</tt></b>' representing the (zero based) absolute index. <b><tt>n</tt></b> is typically larger than 0 because the first coupler has that address.
      | 
      | <li> SSId addressing: the Secondary Slave Addressing has the form '<b><tt>#s:n</tt></b>' where <b><tt>s</tt></b> is the Secondary Slave Id of the EtherCAT coupler and <b><tt>n</tt></b> is the offset in that field. The SSId has to be preprogrammed into the coupler with other service tools.
      | </ol>
      | 
      | <h4>EtherCATInfo XML File:</h4>
      | A string path pointing to the XML description of the k-Bus Coupler
      | 
      | <h4>Sample Time:</h4>
      | Set the <b>Sample Time</b> for the block. <tt>0</tt> is continuous sample time (runs at the model's base rate). Setting <tt>-1</tt> will try to set the time using back propagation.
      mask StyleString: edit,edit,edit,popup(No Grouping|Group Data Types in PDO|Group Data Types),edit
      mask Display:
      | fprintf('BK1120\nK-Bus Coupler\n%s\nM:%s Idx:%s',...
      |     display_name,masterStr,positionStr);
  MSD_0 : S-Function  FunctionName=moog_msd  Parameters=master,index,tsample,iomode  mask(Moog MSC){master=0, index=0, tsample=0, iomode=Inputs and Outputs}
      mask prompts: index "Slave Index"; tsample "Sample Time"; iomode "Input/Output Mode"
      mask help: Moog Servodrive Controller
      mask init:
      | moog_msd_callback('display_callback',gcb)
      mask StyleString: edit,edit,edit,popup(Inputs and Outputs|Inputs only|Outputs only)
      mask CallbackString: |||moog_msd_callback('display_callback',gcb)
      mask Display: fprintf('Moog Servo Drive\nM:%i Idx:%s', master, index) image(imread('moog.png'), [.3, .7, .4, .2]) port_label('input', 1, 'control') port_label('input', 2, 'v_tgt') port_label('output', 1, 'status') port_label('output', 2, 'v_cur')
  Master State : S-Function  FunctionName=master_state  Parameters=master,tsample  mask(Master State){master=0, tsample=0}
      mask prompts: tsample "Sample Time"
      mask help:
      | Outputs master state:
      | * number of responding slaves
      | * Slave states
      | * Link up
      mask Display:
      | fprintf('Master State\nM: %u',
      | master);
  SSI_0 : S-Function  FunctionName=ec_slave2  Parameters=Address,SlaveConfig,LayoutVersion,SdoConfig,output,tsample  mask(EL5001){master=0, index=1, scale=1, offset=0, dtype=Double, code=Binary, baud=1250k, frame=Multiturn (25 bits), fsize=25, length=24, frame_error=off, inhibit=off, inh_time=1, status=off, filter=off, tau=0.1, tsample=0}
      mask prompts: index "Slave Index"; scale "Output Full Scale"; offset "Output Offset"; dtype "Output Data Type"; code "SSI Code"; baud "Baudrate"; frame "Frame Type"; fsize "SSI Frame Size"; length "Data Length"; frame_error "Disable Frame Error"; inhibit "Enable Inhibit Time"; inh_time "Min Inhibit Time [us] (1..65535)"; status "Status Output"; filter "Output Filter"; tau "LPF Time Constant (sec)"; tsample "Sample Time"
      mask help: Beckhoff EtherCAT SSI Input
      mask init:
      | masterStr = '';
      | positionStr = '';
      | [Address masterStr positionStr] = getEtherCATAddress(gcb,master,index);
      | 
      | product_code = hex2dec('13893052');
      | revision_no = hex2dec('00010000');
      | 
      | try 
      |     load EtherCATInfo_el5xxx
      | catch
      |     errordlg([gcb ': Could not load EtherCATInfo MAT file '...
      |         'EtherCATInfo_el5xxx']);
      |     % Regenerate with: 
      |     %  EtherCATInfo_el5xxx = getEtherCATInfo('Beckhoff EL5xxx.xml')
      |     %  save EtherCATInfo_el5xxx 'EtherCATInfo_el5xxx'
      | end
      | 
      | LayoutVersion = 0;
      | SdoConfig = [
      |     hex2dec('4061'), 1,  8, frame_error     ;... % FrameError
      |     hex2dec('4061'), 2,  8, 1               ;... % Power Fail
      |     hex2dec('4061'), 3,  8, inhibit         ;... % Enable Inhibit
      |     hex2dec('4066'), 0,  8, code == 2       ;... % SSI Code
      |     hex2dec('4067'), 0, 16, baud            ;... % Baud Rate
      |     hex2dec('4068'), 0,  8, frame-1         ;... % Frame Type
      |     hex2dec('4069'), 0, 16, fsize           ;... % Frame Size
      |     hex2dec('406A'), 0, 16, length          ;... % Data Length
      |     hex2dec('406B'), 0, 16, inh_time        ;... % Inhibit Time
      |     ];
      | SdoConfig = cell2struct(...
      |     num2cell(SdoConfig),...
      |     {'Index' 'SubIndex' 'BitLen' 'Value'}, 2);
      | 
      | SlaveConfig = genSlaveConfig(EtherCATInfo_el5xxx, product_code, revision_no);
      | 
      | output = [];
      | 
      | if isempty(SlaveConfig.ProductCode)
      |     errordlg(sprintf(...
      |         ['%s: Could not find device with\n'...
      |         'ProductCode \t#x%08X\n'...
      |         'RevisionNo \t#x%08X\n'...
      |         'in file EtherCATInfo_el5xxx.'],...
      |         gcs, product_code, revision_no));
      | else
      |     pdo_entry = [ ...
      |         hex2dec('6000'), 1;...  % Status
      |         hex2dec('6000'), 2];    % Value
      |     
      |     output.PdoEntry = pdo_entry(2,:);
      |     
      |     if dtype ~= 1
      |         output.PdoFullScale = 2^32;
      |         if dtype == 3
      |             output.Gain = scale;
      |             output.Offset = offset;
      |             output.GainName = 'FullScale';
      |             output.OffsetName = 'Offset';
      |         end
      |         if filter
      |             if sum(tau == 0)
      |                 errordlg([gcb ': Specify a nonzero time constant '...
      |                     'for the output filter.']);
      |             end
      |             if (tsample)
      |                 output.Filter = tsample/tau;
      |                 output.FilterName = 'InputWeight';
      |             else
      |                 output.Filter = 2*pi/tau;
      |                 output.FilterName = 'Omega';
      |             end
      |         end
      |     end
      | 
      |     if status
      |         output(2).PdoEntry = pdo_entry(1,:);
      |     end
      | end
      mask Help:
      | This block implements the EtherCAT SSI Input Terminal EL5001.
      | 
      | The first output is data, the second optional output is a Status Byte. Various options affect the behaviour of the terminal and the block's output:
      | 
      | <h4>Master:</h4>
      | Set the EtherCAT Master of this terminal.
      | 
      | <h4>Slave Index:</h4>
      | Set the EtherCAT slave index. Following address formats are allowed:
      | <ol>
      | <li> Absolute addressing: a number <<b><tt>n</tt></b>> representing the (zero based) absolute index. <b><tt>n</tt></b> is typically larger than 0 because the first coupler has that address.
      | 
      | <li> SSId addressing: the Secondary Slave Addressing has the form <<b><tt>#s:n</tt></b>> where <b><tt>s</tt></b> is the Secondary Slave Id of the EtherCAT coupler and <b><tt>n</tt></b> is the offset in that field. The SSId has to be preprogrammed into the coupler with other service tools.
      | </ol>
      | 
      | <h4>Output Full Scale</h4>
      | When <b>Output Data Type</b> is set to <b>Double with scale and offset</b>, the block's output value at full scale terminal input can be set here. This value  directly affects the output despite a possible output LPF filter.
      | 
      | <h4>Output Offset</h4>
      | When <b>Output Data Type</b> is set to <b>Double with scale and offset</b>, the blocks output at zero terminal input can be set here. Note that the Full Scale above is also increased by this amount. This value  directly affects the output despite a possible output LPF filter.
      | 
      | <h4>Output Data Type</h4>
      | Choose the block's output data type for the output signal. Available are:
      | <ul>
      | <li><b><tt>Raw</tt></b> outputting the internal raw value as <tt>uint32_T</tt> as appropriate
      | <li><b><tt>Double</tt></b> outputting 0..1 corresponding to the Full Scale. Full Scale is affected by the Frame Type, SSI Frame Size and Data Length. Refer to manufactuer's documentation.
      | <li><b><tt>Double with scale and offset</tt></b>, allowing the output to be scaled with an offset.
      | </ul>
      | 
      | <p>
      | For <b>SSI Code</b>, <b>Baudrate</b>, <b>Frame Type</b>, <b>SSI Frame Size</b>, <b>Data Length</b>, <b>Disable Frame Error</b>, <b>Enable Inhibit Time</b> and <b>Min Inhibit Time</b>, refer to manufacturer's documentation.
      | <p>
      | Choosing <b>Status Output</b> provides a port of type <tt>uint8_T</tt> where the status is presented. Refer to manufacturors documentation for the used coding.
      | 
      | <h4>Output Filter</h4>
      | When not in <b>Raw</b> mode, the <b>Output Filter</b> checkbox becomes available, allowing the use of an internal low pass filter. Enter the <b>LPF Time Constant</b> for the filter in the field below.
      | <br>For continuous sample time systems (0 in Sample Time), the filter is also continuous. Discrete samples systems (Sample Time > 0) uses an equivalent discrete low pass filter with a similar time constant.
      | 
      | <p>
      | Set the <b>Sample Time</b> for the block. <tt>0</tt> is continuous sample time (runs at the model's base rate). Setting <tt>-1</tt> will try to set the time using back propagation.
      mask StyleString: edit,edit,edit,edit,popup(Raw bits|Double|Double with scale and offset),popup(Binary|Gray),popup(1250k|1000k|500k|250k|125k),popup(Multiturn (25 bits)|Singleturn (13 bits)|Variable (set size in Frame Size)),popup(1|2|3|4|5|6|7|8|9|10|11|12|13|14|15|16|17|18|19|20|21|22|23|24|25|26|27|28|29|30|31|32),popup(1|2|3|4|5|6|7|8|9|10|11|12|13|14|15|16|17|18|19|20|21|22|23|24|25|26|27|28|29|30|31|32),checkbox,checkbox,edit,checkbox,checkbox,edit,edit
      mask CallbackString: ||||el5001_check('dtype');|||el5001_check('frame');||||el5001_check('inhibit');|el5001_check('inh_time');||el5001_check('filter');||
      mask Display:
      | fprintf('EL5001\nSSI Input\nM:%s Idx:%s',...
      |     masterStr,positionStr)
